simulink model "codegen_arm_webots"  (R2025b)
settings: Solver=FixedStepAuto  StartTime=0.0  StopTime=10.0  FixedStep=0.001  RelTol=1e-3
libraries: simulink x1, aerolibguid x1
settings Model: Creator=rowan  LastModifiedBy=rowan
settings OptimizationCC: DefaultParameterBehavior=Inlined  UseDivisionForNetSlopeComputation=on  GainParamInheritBuiltInType=on  UseFloatMulNetSlope=on  InlineInvariantSignals=on  PassReuseOutputArgsAs=Individual arguments  ZeroExternalMemoryAtStartup=off  ZeroInternalMemoryAtStartup=off  NoFixptDivByZeroProtection=on  EfficientFloat2IntCast=on  LifeSpan=1  OptimizeBlockOrder=speed  DifferentSizesBufferReuse=on  EfficientTunableParamExpr=on
settings DebuggingCC: ParameterTunabilityLossMsg=error
settings HardwareCC: ProdBitPerLong=64.0  ProdLongLongMode=on  ProdHWDeviceType=Intel->x86-64 (Linux 64)
settings SFSimCC: MATLABDynamicMemAlloc=off
settings RTWCC: SystemTargetFile=ert.tlc  TemplateMakefile=ert_default_tmf  Description=Embedded Coder
settings CodeAppCC: ForceParamTrailComments=on  IgnoreCustomStorageClasses=off  OperatorAnnotations=on  SimulinkDataObjDesc=on  SFDataObjDesc=on  CustomSymbolStrGlobalVar=rt$N$M  CustomSymbolStrType=$N$M  CustomSymbolStrFcn=$N$M$F  CustomSymbolStrMacro=$N$M  InsertBlockDesc=on
settings ERTTargetCC: ERTCustomFileTemplate=example_file_process.tlc  ERTFilePackagingFormat=CompactWithDataFile  TargetLangStandard=C99 (ISO)  GenerateSampleERTMain=on  IncludeMdlTerminateFcn=off  CombineSignalStateStructs=on  SupportAbsoluteTime=off  SupportComplex=off  SupportNonInlinedSFcns=on

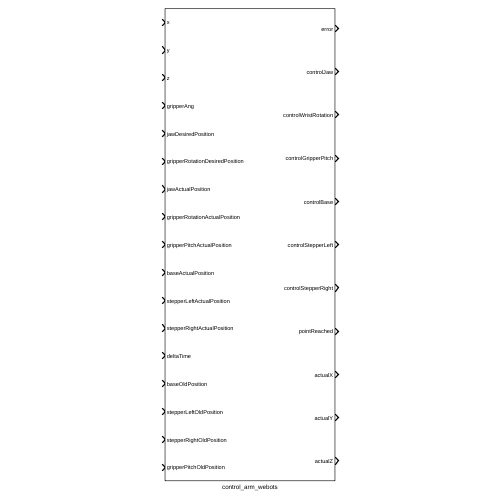
[thumbnail: Simulink's stored preview of the top-level diagram]
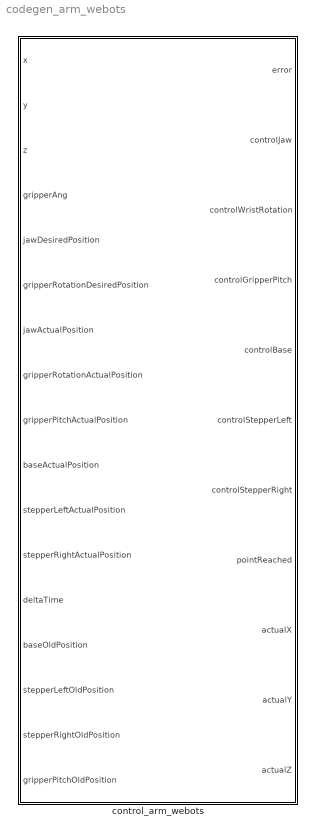
== system codegen_arm_webots ==
  control_arm_webots : Subsystem

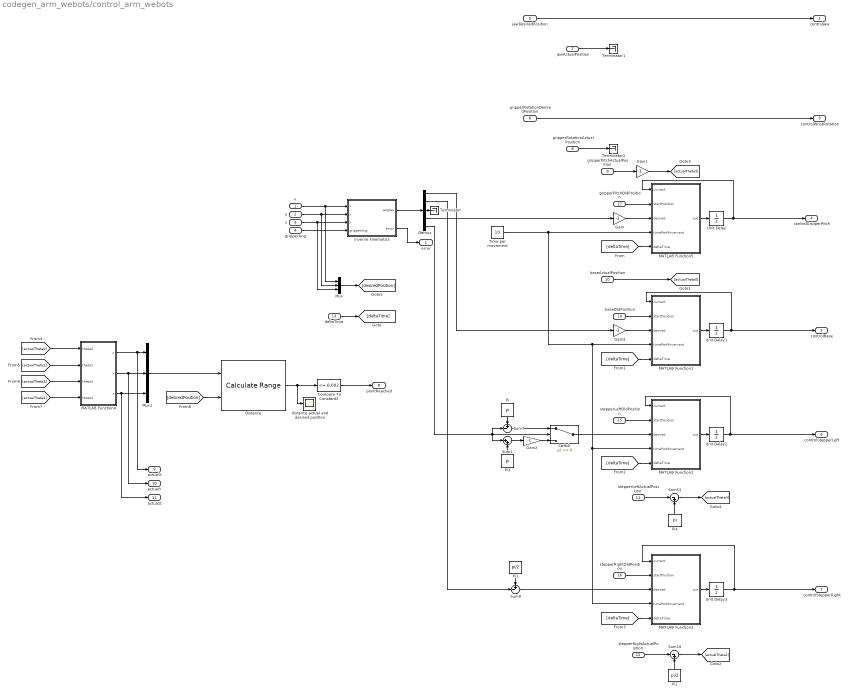
== system codegen_arm_webots/control_arm_webots ==
  x : Inport
  y : Inport  Port=2
  z : Inport  Port=3
  gripperAng : Inport  Port=4
  jawDesiredPosition : Inport  Port=5
  gripperRotationDesiredPosition : Inport  Port=6
  jawActualPosition : Inport  Port=7
  gripperRotationActualPosition : Inport  Port=8
  gripperPitchActualPosition : Inport  Port=9
  baseActualPosition : Inport  Port=10
  stepperLeftActualPosition : Inport  Port=11
  stepperRightActualPosition : Inport  Port=12
  deltaTime : Inport  Port=13
  baseOldPosition : Inport  Port=14
  stepperLeftOldPosition : Inport  Port=15
  stepperRightOldPosition : Inport  Port=16
  gripperPitchOldPosition : Inport  Port=17
  Compare To Constant3 : simulink/Logic and Bit Operations/Compare To Constant  relop=<=  const=0.002  OutDataTypeStr=boolean
  Demux : Demux  Outputs=5
  Distance : aerolibguid/Calculate Range
  Gain{,1..3} (4 alike) : Gain  Gain=-1
  MATLAB Function1 : MATLAB Function  TreatAsAtomicUnit=on
  MATLAB Function2 : MATLAB Function  TreatAsAtomicUnit=on
  MATLAB Function3 : MATLAB Function  TreatAsAtomicUnit=on
  MATLAB Function4 : MATLAB Function  TreatAsAtomicUnit=on
  MATLAB Function5 : MATLAB Function  TreatAsAtomicUnit=on
  Mux : Mux  Inputs=3
  Mux1 : Mux  Inputs=3
  Pi : Constant  Value=pi  OutDataTypeStr=Inherit: Inherit via back propagation
  Pi1 : Constant  Value=pi/2  OutDataTypeStr=Inherit: Inherit via back propagation
  Pi2 : Constant  Value=pi/2  OutDataTypeStr=Inherit: Inherit via back propagation
  Pi3 : Constant  Value=pi  OutDataTypeStr=Inherit: Inherit via back propagation
  Pi4 : Constant  Value=pi  OutDataTypeStr=Inherit: Inherit via back propagation
  Sum1 : Sum  Inputs=|++
  Sum10 : Sum  Inputs=|-+
  Sum11 : Sum  Inputs=|-+
  Sum7 : Sum  Inputs=+-|
  Sum9 : Sum  Inputs=+-|
  Switch : Switch  SaturateOnIntegerOverflow=off  InputSameDT=off
  Terminator : Terminator
  Terminator1 : Terminator
  Terminator2 : Terminator
  Time per movement : Constant  Value=10
  Unit Delay{,1..3} (4 alike) : UnitDelay  SampleTime=-1  HasFrameUpgradeWarning=on
  distance actual and desired position : Scope
      settings: ActiveDisplayYMinimum=-0.023965726590782978  ActiveDisplayYMaximum=0.067046767359712087  DataLoggingVariableName=ScopeData12
  inverse kinematics : MATLAB Function  TreatAsAtomicUnit=on
  error : Outport
  controlJaw : Outport  Port=2
  controlWristRotation : Outport  Port=3
  controlGripperPitch : Outport  Port=4
  controlBase : Outport  Port=5
  controlStepperLeft : Outport  Port=6
  controlStepperRight : Outport  Port=7
  pointReached : Outport  Port=8
  actualX : Outport  Port=9
  actualY : Outport  Port=10
  actualZ : Outport  Port=11
  wires:
  stepperLeftActualPosition/1 -> Sum11/1
  Sum9/1 -> MATLAB Function3/3(desired)
  gripperPitchActualPosition/1 -> Gain1/1
  stepperRightActualPosition/1 -> Sum10/1
  x/1 -> Mux/1, inverse kinematics/1(x)
  y/1 -> inverse kinematics/2(y), Mux/2
  z/1 -> inverse kinematics/3(z), Mux/3
  Demux/5 -> Sum1/1, Sum7/2, Switch/2
  Demux/2 -> Sum9/2
  gripperAng/1 -> inverse kinematics/4(gripperAng)
  Demux/1 -> Gain3/1
  Demux/4 -> Gain/1
  inverse kinematics/2(error) -> error/1
  inverse kinematics/1(angles) -> Demux/1
  deltaTime/1 -> [deltaTime]
  Pi/1 -> Sum7/1
  Pi1/1 -> Sum9/1
  Demux/3 -> Terminator/1
  Mux/1 -> [desiredPosition]
  MATLAB Function4/3(z) -> actualZ/1, Mux1/3
  Pi2/1 -> Sum10/2
  [desiredPosition] -> Distance/2
  Compare To Constant3/1 -> pointReached/1
  [actualTheta3] -> MATLAB Function4/3(theta3)
  MATLAB Function4/2(y) -> actualY/1, Mux1/2
  Distance/1 -> Compare To Constant3/1, distance actual and desired position/1
  MATLAB Function4/1(x) -> actualX/1, Mux1/1
  [actualTheta0] -> MATLAB Function4/1(theta0)
  Mux1/1 -> Distance/1
  gripperRotationDesiredPosition/1 -> controlWristRotation/1
  gripperRotationActualPosition/1 -> Terminator2/1
  Pi4/1 -> Sum11/2
  [actualTheta1] -> MATLAB Function4/2(theta1)
  [actualTheta4] -> MATLAB Function4/4(theta4)
  Sum11/1 -> [actualTheta4]
  Sum10/1 -> [actualTheta1]
  Gain/1 -> MATLAB Function5/3(desired)
  Gain1/1 -> [actualTheta3]
  baseActualPosition/1 -> [actualTheta0]
  Gain3/1 -> MATLAB Function1/3(desired)
  Switch/1 -> MATLAB Function2/3(desired)
  Sum7/1 -> Switch/1
  Pi3/1 -> Sum1/2
  Sum1/1 -> Gain2/1
  Gain2/1 -> Switch/3
  jawActualPosition/1 -> Terminator1/1
  jawDesiredPosition/1 -> controlJaw/1
  gripperPitchOldPosition/1 -> MATLAB Function5/2(startPosition)
  Time per movement/1 -> MATLAB Function5/4(timePerMovement), MATLAB Function3/4(timePerMovement), MATLAB Function2/4(timePerMovement), MATLAB Function1/4(timePerMovement)
  [deltaTime] -> MATLAB Function5/5(deltaTime)
  MATLAB Function5/1(out) -> Unit Delay/1
  MATLAB Function1/1(out) -> Unit Delay1/1
  baseOldPosition/1 -> MATLAB Function1/2(startPosition)
  [deltaTime] -> MATLAB Function1/5(deltaTime)
  stepperLeftOldPosition/1 -> MATLAB Function2/2(startPosition)
  MATLAB Function2/1(out) -> Unit Delay2/1
  [deltaTime] -> MATLAB Function2/5(deltaTime)
  Unit Delay/1 -> controlGripperPitch/1, MATLAB Function5/1(current)
  Unit Delay1/1 -> MATLAB Function1/1(current), controlBase/1
  Unit Delay2/1 -> MATLAB Function2/1(current), controlStepperLeft/1
  MATLAB Function3/1(out) -> Unit Delay3/1
  stepperRightOldPosition/1 -> MATLAB Function3/2(startPosition)
  [deltaTime] -> MATLAB Function3/5(deltaTime)
  Unit Delay3/1 -> MATLAB Function3/1(current), controlStepperRight/1

== matlab function codegen_arm_webots/control_arm_webots/MATLAB Function1 ==
  data: current input; startPosition input; out output; desired input; timePerMovement input; deltaTime input
function out = linear_interpolation(current, startPosition, desired, timePerMovement, deltaTime)

velocity = abs(desired - startPosition) / timePerMovement;

if current < desired
    current = current + (velocity * deltaTime);
end
if current > desired
    current = current - (velocity * deltaTime);
end
%setting final position if it is close
if abs(current - desired) < 0.01
    current = desired;
end


out = current;

== matlab function codegen_arm_webots/control_arm_webots/inverse kinematics ==
  data: x input; angles output; y input; z input; gripperAng input; error output
function [angles, error] = IK(x, y, z, gripperAng)
    alpha = gripperAng;
    defaultAngles = [0; pi/2; 0; 0; pi];
    
    %all the lengths are in meters
    LbaseToP1 = 0.065;
    LbaseToP3 = 0.149;
    
    LP1toP2 = 0.350;
    LP2toP6 = 0.500;
    LP6toP7 = 0.300;
    
    LP3toP4 = 0.120;
    LP4toP5 = 0.280;
    LP5toP2 = 0.120;
    
    if x < 0
        theta0 = atan(y/x) + pi;
    else
        theta0 = atan(y/x);
    end
    angToBase = theta0 - pi;

    if theta0 > pi
        theta0 = theta0 - 2*pi;
    end

    theta0 = theta0 * -1;
    
    %setting end position, rotated towards the base
    P7i = [cos(angToBase) -sin(angToBase) 0 x;
           sin(angToBase)  cos(angToBase) 0 y;
           0               0              1 z;
           0               0              0 1];
    
    %rotation x
    P7i = P7i * [1 0  0 0;
                 0 0 -1 0;
                 0 1  0 0;
                 0 0  0 1];
    
    %rotation z
    TP7toP6i = [cos(alpha) -sin(alpha) 0 0;
                sin(alpha)  cos(alpha) 0 0;
                0           0          1 0;
                0           0          0 1];
    
    %translation x
    TP7toP6i = TP7toP6i * [1 0 0 LP6toP7;
                           0 1 0  0;
                           0 0 1  0;
                           0 0 0  1];
    
    P6i = P7i * TP7toP6i;
    
    %translation z
    P1i = [1 0 0 0;
           0 1 0 0;
           0 0 1 LbaseToP1;
           0 0 0 1];
    
    
    %calculating theta1, theta2 and theta3
    L_1i = LP1toP2; L_2i = LP2toP6;
    dx = P6i(1,4) - P1i(1,4);
    dy = P6i(2,4) - P1i(2,4);
    XEi = sqrt(dx*dx + dy*dy);
    YEi = P6i(3,4) - P1i(3,4);
    
    if (- L_1i^4 + 2*L_1i^2*L_2i^2 + 2*L_1i^2*XEi^2 + 2*L_1i^2*YEi^2 - L_2i^4 + 2*L_2i^2*XEi^2 + 2*L_2i^2*YEi^2 - XEi^4 - 2*XEi^2*YEi^2 - YEi^4) < 0
        angles = defaultAngles;
        error = 1;
        return;
    end

    theta1 = 2*atan((2*L_1i*YEi + sqrt(- L_1i^4 + 2*L_1i^2*L_2i^2 + 2*L_1i^2*XEi^2 + 2*L_1i^2*YEi^2 - L_2i^4 + 2*L_2i^2*XEi^2 + 2*L_2i^2*YEi^2 - XEi^4 - 2*XEi^2*YEi^2 - YEi^4))/(L_1i^2 + 2*L_1i*XEi - L_2i^2 + XEi^2 + YEi^2));
    theta2 = -2*atan(sqrt((- L_1i^2 + 2*L_1i*L_2i - L_2i^2 + XEi^2 + YEi^2)*(L_1i^2 + 2*L_1i*L_2i + L_2i^2 - XEi^2 - YEi^2))/(- L_1i^2 + 2*L_1i*L_2i - L_2i^2 + XEi^2 + YEi^2));
    
    theta3 = -alpha -theta1 -theta2;
    
    
    %getting currently known transforms
    %{ 
    commented out transforms are only used for forward kinematics
    %rotation z
    TP0toPbase = [cos(theta0) -sin(theta0) 0 0;
                  sin(theta0)  cos(theta0) 0 0;
                  0            0           1 0;
                  0            0           0 1];
    %}
    
    %translation z then rotation x
    TPbasetoP1 = [1 0 0  0;
                  0 0 -1 0;
                  0 1 0  LbaseToP1;
                  0 0 0  1];
    %rotation z
    TPbasetoP1 = TPbasetoP1 * [cos(theta1) -sin(theta1) 0 0;
                               sin(theta1)  cos(theta1) 0 0;
                               0            0           1 0;
                               0            0           0 1];
    
    %translation x then rotation z
    TP1toP2 = [cos(theta2) -sin(theta2) 0 LP1toP2;
               sin(theta2)  cos(theta2) 0 0;
               0            0           1 0;
               0            0           0 1];
    
    %{
    %translation x then rotation z
    TP2toP6 = [cos(theta3) -sin(theta3) 0 LP2toP6;
               sin(theta3)  cos(theta3) 0 0;
               0            0           1 0;
               0            0           0 1];
    
    %translation x
    TP6toP7 = [1 0 0 LP6toP7;
               0 1 0 0;
               0 0 1 0;
               0 0 0 1];
    %}    

    %translation z then rotation x
    TPbasetoP3 = [1 0 0  0;
                  0 0 -1 0;
                  0 1 0  LbaseToP3;
                  0 0 0  1];
    
    %translation x
    TP2toP5 = [1 0 0 -LP5toP2;
               0 1 0 0;
               0 0 1 0;
               0 0 0 1];
    
    %initial position
    P0 = [1 0 0 0;
          0 1 0 0;
          0 0 1 0;
          0 0 0 1];
    
    %{
    %translation x
    TP4toP5 = [1 0 0 LP4toP5;
               0 1 0 0;
               0 0 1 0;
               0 0 0 1];
    %}
    
    %getting position for paralellagram angles
    P3planar = P0 * TPbasetoP3;
    P5planar = P0 * TPbasetoP1 * TP1toP2 * TP2toP5;
    
    %getting parallelageram angles
    L_1 = LP3toP4; L_2 = LP4toP5;
    XE = P5planar(1, 4) - P3planar(1, 4);
    YE = P5planar(3, 4) - P3planar(3, 4);
    theta4 = 2*atan((2*L_1*YE + sqrt(- L_1^4 + 2*L_1^2*L_2^2 + 2*L_1^2*XE^2 + 2*L_1^2*YE^2 - L_2^4 + 2*L_2^2*XE^2 + 2*L_2^2*YE^2 - XE^4 - 2*XE^2*YE^2 - YE^4))/(L_1^2 + 2*L_1*XE - L_2^2 + XE^2 + YE^2));
    %theta5 = -2*atan(sqrt((- L_1^2 + 2*L_1*L_2 - L_2^2 + XE^2 + YE^2)*(L_1^2 + 2*L_1*L_2 + L_2^2 - XE^2 - YE^2))/(- L_1^2 + 2*L_1*L_2 - L_2^2 + XE^2 + YE^2));
    
    
    %getting the last transforms
    %{
    %rotation z
    TPbasetoP3 = TPbasetoP3 * [cos(theta4) -sin(theta4) 0 0;
                               sin(theta4)  cos(theta4) 0 0;
                               0            0           1 0;
                               0            0           0 1];
    
    %translation x then rotation z
    TP3toP4 = [cos(theta5) -sin(theta5) 0 LP3toP4;
               sin(theta5)  cos(theta5) 0 0;
               0            0           1 0;
               0            0           0 1];
    %}
    
    %{
    this is being problematic at the moment
    if (abs(theta0) > pi) || (theta1 < 0) || (theta1 > 3/4*pi) || (theta3 < -3/4*pi) || (theta3 > pi/4) || (theta4 < pi/2) || (theta4 > 3/2*pi)
        angles = defaultAngles;
        error = 2;
        return;
    end
    %}
    
    %passing the angles to the output
    angles = [theta0; theta1; theta2; theta3; theta4];
    error = 0;
    return;
end

== matlab function codegen_arm_webots/control_arm_webots/MATLAB Function2 ==
  data: current input; startPosition input; out output; desired input; timePerMovement input; deltaTime input
function out = linear_interpolation(current, startPosition, desired, timePerMovement, deltaTime)

velocity = abs(desired - startPosition) / timePerMovement;

if current < desired
    current = current + (velocity * deltaTime);
end
if current > desired
    current = current - (velocity * deltaTime);
end
%setting final position if it is close
if abs(current - desired) < 0.01
    current = desired;
end

out = current;

== matlab function codegen_arm_webots/control_arm_webots/MATLAB Function3 ==
  data: current input; startPosition input; out output; desired input; timePerMovement input; deltaTime input
function out = linear_interpolation(current, startPosition, desired, timePerMovement, deltaTime)

velocity = abs(desired - startPosition) / timePerMovement;

if current < desired
    current = current + (velocity * deltaTime);
end
if current > desired
    current = current - (velocity * deltaTime);
end
%setting final position if it is close
if abs(current - desired) < 0.01
    current = desired;
end

out = current;

== matlab function codegen_arm_webots/control_arm_webots/MATLAB Function4 ==
  data: x output; theta0 input; y output; z output; theta1 input; theta3 input; theta4 input
function [x, y, z] = FK(theta0, theta1, theta3, theta4)
    %defining dimentions
    LbaseToP1 = 0.065;
    LbaseToP3 = 0.149;

    LP1toP2 = 0.350;
    LP5toP6 = 0.620;
    LP5toP2 = 0.120;
    LP6toP7 = 0.300;

    LP3toP4 = 0.120;
    LP4toP5 = 0.280;

    %rotation z
    TP0toPbase = [cos(theta0) -sin(theta0) 0 0;
                  sin(theta0)  cos(theta0) 0 0;
                  0            0           1 0;
                  0            0           0 1];

    %translation z then rotation x
    TPbasetoP1 = [1 0 0  0;
                  0 0 -1 0;
                  0 1 0  LbaseToP1;
                  0 0 0  1];

    %rotation z
    TPbasetoP1 = TPbasetoP1 * [cos(theta1) -sin(theta1) 0 0;
                               sin(theta1)  cos(theta1) 0 0;
                               0            0           1 0;
                               0            0           0 1];

    %translation x
    TP1toP2 = [1 0 0 LP1toP2;
               0 1 0 0;
               0 0 1 0;
               0 0 0 1];

    %translation x then rotation z
    TP5toP6 = [cos(theta3) -sin(theta3) 0 LP5toP6;
               sin(theta3)  cos(theta3) 0 0;
               0            0           1 0;
               0            0           0 1];

    %translation x
    TP6toP7 = [1 0 0 LP6toP7;
               0 1 0 0;
               0 0 1 0;
               0 0 0 1];

    %translation z then rotation x
    TPbasetoP3 = [1 0  0 0;
                  0 0 -1 0;
                  0 1  0 LbaseToP3;
                  0 0  0 1];

    %translation x
    TP3toP4 = [1 0 0 LP3toP4;
               0 1 0 0;
               0 0 1 0;
               0 0 0 1];

    %rotation z
    TPbasetoP3 = TPbasetoP3 * [cos(theta4) -sin(theta4) 0 0;
                               sin(theta4)  cos(theta4) 0 0;
                               0            0           1 0;
                               0            0           0 1];

    %initial position
    P0 = [1 0 0 0;
          0 1 0 0;
          0 0 1 0;
          0 0 0 1];

    %getting position for paralellagram angles
    P2planar = P0 * TPbasetoP1 * TP1toP2;
    P4planar = P0 * TPbasetoP3 * TP3toP4;

    L_1 = LP4toP5; L_2 = LP5toP2;
    XE = P4planar(1, 4) - P2planar(1, 4);
    YE = P4planar(3, 4) - P2planar(3, 4);
    if (- L_1^4 + 2*L_1^2*L_2^2 + 2*L_1^2*XE^2 + 2*L_1^2*YE^2 - L_2^4 + 2*L_2^2*XE^2 + 2*L_2^2*YE^2 - XE^4 - 2*XE^2*YE^2 - YE^4) > 0
        theta5 = 2*atan((2*L_1*YE + sqrt(- L_1^4 + 2*L_1^2*L_2^2 + 2*L_1^2*XE^2 + 2*L_1^2*YE^2 - L_2^4 + 2*L_2^2*XE^2 + 2*L_2^2*YE^2 - XE^4 - 2*XE^2*YE^2 - YE^4))/(L_1^2 + 2*L_1*XE - L_2^2 + XE^2 + YE^2));
        theta6 = -2*atan(sqrt((- L_1^2 + 2*L_1*L_2 - L_2^2 + XE^2 + YE^2)*(L_1^2 + 2*L_1*L_2 + L_2^2 - XE^2 - YE^2))/(- L_1^2 + 2*L_1*L_2 - L_2^2 + XE^2 + YE^2));
    else
        theta5 = 0;
        theta6 = 0;
    end

    theta5 = theta5+(pi-theta4);

    %translation x then rotation z
    TP3toP4 = [cos(theta5) -sin(theta5) 0 LP3toP4;
               sin(theta5)  cos(theta5) 0 0;
               0            0           1 0;
               0            0           0 1];

    %translation x then rotation z
    TP4toP5 = [cos(theta6) -sin(theta6) 0 LP4toP5;
               sin(theta6)  cos(theta6) 0 0;
               0            0           1 0;
               0            0           0 1];

    Pbase = TP0toPbase;
    P3 = Pbase * TPbasetoP3;
    P4 = P3 * TP3toP4;
    P5 = P4 * TP4toP5;
    P6 = P5 * TP5toP6;
    P7 = P6 * TP6toP7;

    x = P7(1,4);
    y = P7(2,4);
    z = P7(3,4);
end

== matlab function codegen_arm_webots/control_arm_webots/MATLAB Function5 ==
  data: current input; startPosition input; out output; desired input; timePerMovement input; deltaTime input
function out = linear_interpolation(current, startPosition, desired, timePerMovement, deltaTime)

velocity = abs(desired - startPosition) / timePerMovement;

if current < desired
    current = current + (velocity * deltaTime);
end
if current > desired
    current = current - (velocity * deltaTime);
end
%setting final position if it is close
if abs(current - desired) < 0.01
    current = desired;
end

out = current;
